simulink model "SAME5x_PIM_MCLV2_Test_programme_2020a"  (Simulink 10.1)
(part 2 of 2)

      mask TypeOptions FDMTEN: Deadman Timer is enabled | Deadman Timer is disabled
      mask TypeOptions TRCEN: Trace features in the CPU are enabled | Trace features in the CPU are disabled
      mask TypeOptions BOOTISA: Boot code and Exception code is MIPS32 | Boot code and Exception code is microMIPS
      mask TypeOptions FECCCON: ECC and Dynamic ECC are disabled (ECCCON<1:0> bits are writable) | ECC and Dynamic ECC are disabled (ECCCON<1:0> bits are locked) | Dynamic Flash ECC is enabled (ECCCON<1:0> bits are locked) | Flash ECC is enabled (ECCCON<1:0> bits are locked; disables word Flash writes) | ECC and Dynamic ECC are disabled (ECCCON bits are writable) | ECC and Dynamic ECC are disabled (ECCCON bits are locked) | Dynamic Flash ECC is enabled (ECCCON bits are locked) | Flash ECC is enabled (ECCCON bits are locked)
      mask TypeOptions EXTDDRSIZE: Not used
      mask TypeOptions FSLEEP: Flash is powered down when the device is in Sleep mode | Flash power down is controlled by the VREGS bit
      mask TypeOptions DBGPER: Allow CPU access to all permission regions | PG0: Deny PG1: Allow PG2: Allow | PG0: Allow PG1: Deny PG2: Allow | Allow CPU access to Permission Group 2 permission regions | PG0: Allow PG1: Allow PG2: Deny | Allow CPU access to Permission Group 1 permission regions | Allow CPU access to Permission Group 0 permission regions | Deny CPU access to all permission regions
      mask TypeOptions EJTAGBEN: Normal EJTAG functionality | Reduced EJTAG functionality
      mask TypeOptions TSEQ: Not used
      mask TypeOptions CSEQ: Not used
      mask TypeOptions RWDTPS: 1:1048576 | 1:524288 | 1:262144 | 1:131072 | 1:65536 | 1:32768 | 1:16384 | 1:8192 | 1:4096 | 1:2048 | 1:1024 | 1:512 | 1:256 | 1:128 | 1:64 | 1:32 | 1:16 | 1:8 | 1:4 | 1:2 | 1:1 | 1:2147483648 | 1:1073741824 | 1:536870912 | 1:268435456 | 1:134217728 | 1:67108864 | 1:33554432 | 1:16777216 | 1:8388608 | 1:4194304 | 1:2097152
      mask TypeOptions RCLKSEL: Always use LPRC | Use FRC when WINDIS = 0; system clock is not INTOSC/LPRC and device is not in Sleep;otherwise; use INTOSC/LPRC | Use peripheral clk when system clock is not INTOSC/LPRC and device is not in Sleep;otherwise; use INTOSC/LPRC | Always use BFRC/256 | Use FRC when WINDIS = 0 and device is not in Sleep; otherwise; use BFRC/256 | Use peripheral clk when device is not in Sleep; otherwise; use BFRC/256
      mask TypeOptions SWDTPS: 1:1048576 | 1:524288 | 1:262144 | 1:131072 | 1:65536 | 1:32768 | 1:16384 | 1:8192 | 1:4096 | 1:2048 | 1:1024 | 1:512 | 1:256 | 1:128 | 1:64 | 1:32 | 1:16 | 1:8 | 1:4 | 1:2 | 1:1 | 1:2147483648 | 1:1073741824 | 1:536870912 | 1:268435456 | 1:134217728 | 1:67108864 | 1:33554432 | 1:16777216 | 1:8388608 | 1:4194304 | 1:2097152
      mask TypeOptions DMTIVTL: Not used
      mask TypeOptions DMTIVTH: Not used
      mask TypeOptions DMTCNTL: Not used
      mask TypeOptions DMTCNTH: Not used
      mask TypeOptions DMTDIS: Dead Man Timer is Disabled and can be enabled by software | Dead Man Timer is Enabled and cannot be disabled by software
      mask TypeOptions SMBEN: SMBus input threshold is enabled | Standard I2C input threshold operation
      mask TypeOptions SPI2PIN: SPI2 uses I/O remap (PPS) pins | SPI2 uses dedicated I/O pins
      mask TypeOptions CTXT3: Not Assigned | Alternate Register set assigned to IPL level 7 | Alternate Register set assigned to IPL level 6 | Alternate Register set assigned to IPL level 5 | Alternate Register set assigned to IPL level 4 | Alternate Register set assigned to IPL level 3 | Alternate Register set assigned to IPL level 2 | Alternate Register set assigned to IPL level 1
      mask TypeOptions CTXT4: Not Assigned | Alternate Register set assigned to IPL level 7 | Alternate Register set assigned to IPL level 6 | Alternate Register set assigned to IPL level 5 | Alternate Register set assigned to IPL level 4 | Alternate Register set assigned to IPL level 3 | Alternate Register set assigned to IPL level 2 | Alternate Register set assigned to IPL level 1
      mask TypeOptions MBXM0: Mailbox register configured for Master data read (Slave to Master data transfer) | Mailbox register configured for Master data write (Master to Slave data transfer)
      mask TypeOptions MBXM1: Mailbox register configured for Master data read (Slave to Master data transfer) | Mailbox register configured for Master data write (Master to Slave data transfer)
      mask TypeOptions MBXM2: Mailbox register configured for Master data read (Slave to Master data transfer) | Mailbox register configured for Master data write (Master to Slave data transfer)
      mask TypeOptions MBXM3: Mailbox register configured for Master data read (Slave to Master data transfer) | Mailbox register configured for Master data write (Master to Slave data transfer)
      mask TypeOptions MBXM4: Mailbox register configured for Master data read (Slave to Master data transfer) | Mailbox register configured for Master data write (Master to Slave data transfer)
      mask TypeOptions MBXM5: Mailbox register configured for Master data read (Slave to Master data transfer) | Mailbox register configured for Master data write (Master to Slave data transfer)
      mask TypeOptions MBXM6: Mailbox register configured for Master data read (Slave to Master data transfer) | Mailbox register configured for Master data write (Master to Slave data transfer)
      mask TypeOptions MBXM7: Mailbox register configured for Master data read (Slave to Master data transfer) | Mailbox register configured for Master data write (Master to Slave data transfer)
      mask TypeOptions MBXM8: Mailbox register configured for Master data read (Slave to Master data transfer) | Mailbox register configured for Master data write (Master to Slave data transfer)
      mask TypeOptions MBXM9: Mailbox register configured for Master data read (Slave to Master data transfer) | Mailbox register configured for Master data write (Master to Slave data transfer)
      mask TypeOptions MBXM10: Mailbox register configured for Master data read (Slave to Master data transfer) | Mailbox register configured for Master data write (Master to Slave data transfer)
      mask TypeOptions MBXM11: Mailbox register configured for Master data read (Slave to Master data transfer) | Mailbox register configured for Master data write (Master to Slave data transfer)
      mask TypeOptions MBXM12: Mailbox register configured for Master data read (Slave to Master data transfer) | Mailbox register configured for Master data write (Master to Slave data transfer)
      mask TypeOptions MBXM13: Mailbox register configured for Master data read (Slave to Master data transfer) | Mailbox register configured for Master data write (Master to Slave data transfer)
      mask TypeOptions MBXM14: Mailbox register configured for Master data read (Slave to Master data transfer) | Mailbox register configured for Master data write (Master to Slave data transfer)
      mask TypeOptions MBXM15: Mailbox register configured for Master data read (Slave to Master data transfer) | Mailbox register configured for Master data write (Master to Slave data transfer)
      mask TypeOptions MBXHSA: MSIxMBXD15 assigned to mailbox handshake protocol block A | MSIxMBXD14 assigned to mailbox handshake protocol block A | MSIxMBXD13 assigned to mailbox handshake protocol block A | MSIxMBXD12 assigned to mailbox handshake protocol block A | MSIxMBXD11 assigned to mailbox handshake protocol block A | MSIxMBXD10 assigned to mailbox handshake protocol block A | MSIxMBXD9 assigned to mailbox handshake protocol block A | MSIxMBXD8 assigned to mailbox handshake protocol block A | MSIxMBXD7 assigned to mailbox handshake protocol block A | MSIxMBXD6 assigned to mailbox handshake protocol block A | MSIxMBXD5 assigned to mailbox handshake protocol block A | MSIxMBXD4 assigned to mailbox handshake protocol block A | MSIxMBXD3 assigned to mailbox handshake protocol block A | MSIxMBXD2 assigned to mailbox handshake protocol block A | MSIxMBXD1 assigned to mailbox handshake protocol block A | MSIxMBXD0 assigned to mailbox handshake protocol block A
      mask TypeOptions MBXHSB: MSIxMBXD15 assigned to mailbox handshake protocol block B | MSIxMBXD14 assigned to mailbox handshake protocol block B | MSIxMBXD13 assigned to mailbox handshake protocol block B | MSIxMBXD12 assigned to mailbox handshake protocol block B | MSIxMBXD11 assigned to mailbox handshake protocol block B | MSIxMBXD10 assigned to mailbox handshake protocol block B | MSIxMBXD9 assigned to mailbox handshake protocol block B | MSIxMBXD8 assigned to mailbox handshake protocol block B | MSIxMBXD7 assigned to mailbox handshake protocol block B | MSIxMBXD6 assigned to mailbox handshake protocol block B | MSIxMBXD5 assigned to mailbox handshake protocol block B | MSIxMBXD4 assigned to mailbox handshake protocol block B | MSIxMBXD3 assigned to mailbox handshake protocol block B | MSIxMBXD2 assigned to mailbox handshake protocol block B | MSIxMBXD1 assigned to mailbox handshake protocol block B | MSIxMBXD0 assigned to mailbox handshake protocol block B
      mask TypeOptions MBXHSC: MSIxMBXD15 assigned to mailbox handshake protocol block C | MSIxMBXD14 assigned to mailbox handshake protocol block C | MSIxMBXD13 assigned to mailbox handshake protocol block C | MSIxMBXD12 assigned to mailbox handshake protocol block C | MSIxMBXD11 assigned to mailbox handshake protocol block C | MSIxMBXD10 assigned to mailbox handshake protocol block C | MSIxMBXD9 assigned to mailbox handshake protocol block C | MSIxMBXD8 assigned to mailbox handshake protocol block C | MSIxMBXD7 assigned to mailbox handshake protocol block C | MSIxMBXD6 assigned to mailbox handshake protocol block C | MSIxMBXD5 assigned to mailbox handshake protocol block C | MSIxMBXD4 assigned to mailbox handshake protocol block C | MSIxMBXD3 assigned to mailbox handshake protocol block C | MSIxMBXD2 assigned to mailbox handshake protocol block C | MSIxMBXD1 assigned to mailbox handshake protocol block C | MSIxMBXD0 assigned to mailbox handshake protocol block C
      mask TypeOptions MBXHSD: MSIxMBXD15 assigned to mailbox handshake protocol block D | MSIxMBXD14 assigned to mailbox handshake protocol block D | MSIxMBXD13 assigned to mailbox handshake protocol block D | MSIxMBXD12 assigned to mailbox handshake protocol block D | MSIxMBXD11 assigned to mailbox handshake protocol block D | MSIxMBXD10 assigned to mailbox handshake protocol block D | MSIxMBXD9 assigned to mailbox handshake protocol block D | MSIxMBXD8 assigned to mailbox handshake protocol block D | MSIxMBXD7 assigned to mailbox handshake protocol block D | MSIxMBXD6 assigned to mailbox handshake protocol block D | MSIxMBXD5 assigned to mailbox handshake protocol block D | MSIxMBXD4 assigned to mailbox handshake protocol block D | MSIxMBXD3 assigned to mailbox handshake protocol block D | MSIxMBXD2 assigned to mailbox handshake protocol block D | MSIxMBXD1 assigned to mailbox handshake protocol block D | MSIxMBXD0 assigned to mailbox handshake protocol block D
      mask TypeOptions MBXHSE: MSIxMBXD15 assigned to mailbox handshake protocol block E | MSIxMBXD14 assigned to mailbox handshake protocol block E | MSIxMBXD13 assigned to mailbox handshake protocol block E | MSIxMBXD12 assigned to mailbox handshake protocol block E | MSIxMBXD11 assigned to mailbox handshake protocol block E | MSIxMBXD10 assigned to mailbox handshake protocol block E | MSIxMBXD9 assigned to mailbox handshake protocol block E | MSIxMBXD8 assigned to mailbox handshake protocol block E | MSIxMBXD7 assigned to mailbox handshake protocol block E | MSIxMBXD6 assigned to mailbox handshake protocol block E | MSIxMBXD5 assigned to mailbox handshake protocol block E | MSIxMBXD4 assigned to mailbox handshake protocol block E | MSIxMBXD3 assigned to mailbox handshake protocol block E | MSIxMBXD2 assigned to mailbox handshake protocol block E | MSIxMBXD1 assigned to mailbox handshake protocol block E | MSIxMBXD0 assigned to mailbox handshake protocol block E
      mask TypeOptions MBXHSF: MSIxMBXD15 assigned to mailbox handshake protocol block F | MSIxMBXD14 assigned to mailbox handshake protocol block F | MSIxMBXD13 assigned to mailbox handshake protocol block F | MSIxMBXD12 assigned to mailbox handshake protocol block F | MSIxMBXD11 assigned to mailbox handshake protocol block F | MSIxMBXD10 assigned to mailbox handshake protocol block F | MSIxMBXD9 assigned to mailbox handshake protocol block F | MSIxMBXD8 assigned to mailbox handshake protocol block F | MSIxMBXD7 assigned to mailbox handshake protocol block F | MSIxMBXD6 assigned to mailbox handshake protocol block F | MSIxMBXD5 assigned to mailbox handshake protocol block F | MSIxMBXD4 assigned to mailbox handshake protocol block F | MSIxMBXD3 assigned to mailbox handshake protocol block F | MSIxMBXD2 assigned to mailbox handshake protocol block F | MSIxMBXD1 assigned to mailbox handshake protocol block F | MSIxMBXD0 assigned to mailbox handshake protocol block F
      mask TypeOptions MBXHSG: MSIxMBXD15 assigned to mailbox handshake protocol block G | MSIxMBXD14 assigned to mailbox handshake protocol block G | MSIxMBXD13 assigned to mailbox handshake protocol block G | MSIxMBXD12 assigned to mailbox handshake protocol block G | MSIxMBXD11 assigned to mailbox handshake protocol block G | MSIxMBXD10 assigned to mailbox handshake protocol block G | MSIxMBXD9 assigned to mailbox handshake protocol block G | MSIxMBXD8 assigned to mailbox handshake protocol block G | MSIxMBXD7 assigned to mailbox handshake protocol block G | MSIxMBXD6 assigned to mailbox handshake protocol block G | MSIxMBXD5 assigned to mailbox handshake protocol block G | MSIxMBXD4 assigned to mailbox handshake protocol block G | MSIxMBXD3 assigned to mailbox handshake protocol block G | MSIxMBXD2 assigned to mailbox handshake protocol block G | MSIxMBXD1 assigned to mailbox handshake protocol block G | MSIxMBXD0 assigned to mailbox handshake protocol block G
      mask TypeOptions MBXHSH: MSIxMBXD15 assigned to mailbox handshake protocol block H | MSIxMBXD14 assigned to mailbox handshake protocol block H | MSIxMBXD13 assigned to mailbox handshake protocol block H | MSIxMBXD12 assigned to mailbox handshake protocol block H | MSIxMBXD11 assigned to mailbox handshake protocol block H | MSIxMBXD10 assigned to mailbox handshake protocol block H | MSIxMBXD9 assigned to mailbox handshake protocol block H | MSIxMBXD8 assigned to mailbox handshake protocol block H | MSIxMBXD7 assigned to mailbox handshake protocol block H | MSIxMBXD6 assigned to mailbox handshake protocol block H | MSIxMBXD5 assigned to mailbox handshake protocol block H | MSIxMBXD4 assigned to mailbox handshake protocol block H | MSIxMBXD3 assigned to mailbox handshake protocol block H | MSIxMBXD2 assigned to mailbox handshake protocol block H | MSIxMBXD1 assigned to mailbox handshake protocol block H | MSIxMBXD0 assigned to mailbox handshake protocol block H
      mask TypeOptions HSAEN: Mailbox data flow control handshake protocol block disabled. | Mailbox data flow control handshake protocol block enabled
      mask TypeOptions HSBEN: Mailbox data flow control handshake protocol block disabled. | Mailbox data flow control handshake protocol block enabled
      mask TypeOptions HSCEN: Mailbox data flow control handshake protocol block disabled. | Mailbox data flow control handshake protocol block enabled
      mask TypeOptions HSDEN: Mailbox data flow control handshake protocol block disabled. | Mailbox data flow control handshake protocol block enabled
      mask TypeOptions HSEEN: Mailbox data flow control handshake protocol block disabled. | Mailbox data flow control handshake protocol block enabled
      mask TypeOptions HSFEN: Mailbox data flow control handshake protocol block disabled. | Mailbox data flow control handshake protocol block enabled
      mask TypeOptions HSGEN: Mailbox data flow control handshake protocol block disabled. | Mailbox data flow control handshake protocol block enabled
      mask TypeOptions HSHEN: Mailbox data flow control handshake protocol block disabled. | Mailbox data flow control handshake protocol block enabled
      mask TypeOptions CPRA0: Master core owns pin. | Slave 1 core owns pin.
      mask TypeOptions CPRA1: Master core owns pin. | Slave 1 core owns pin.
      mask TypeOptions CPRA2: Master core owns pin. | Slave 1 core owns pin.
      mask TypeOptions CPRA3: Master core owns pin. | Slave 1 core owns pin.
      mask TypeOptions CPRA4: Master core owns pin. | Slave 1 core owns pin.
      mask TypeOptions CPRB0: Master core owns pin. | Slave 1 core owns pin.
      mask TypeOptions CPRB1: Master core owns pin. | Slave 1 core owns pin.
      mask TypeOptions CPRB2: Master core owns pin. | Slave 1 core owns pin.
      mask TypeOptions CPRB3: Master core owns pin. | Slave 1 core owns pin.
      mask TypeOptions CPRB4: Master core owns pin. | Slave 1 core owns pin.
      mask TypeOptions CPRB5: Master core owns pin. | Slave 1 core owns pin.
      mask TypeOptions CPRB6: Master core owns pin. | Slave 1 core owns pin.
      mask TypeOptions CPRB7: Master core owns pin. | Slave 1 core owns pin.
      mask TypeOptions CPRB8: Master core owns pin. | Slave 1 core owns pin.
      mask TypeOptions CPRB9: Master core owns pin. | Slave 1 core owns pin.
      mask TypeOptions CPRB10: Master core owns pin. | Slave 1 core owns pin.
      mask TypeOptions CPRB11: Master core owns pin. | Slave 1 core owns pin.
      mask TypeOptions CPRB12: Master core owns pin. | Slave 1 core owns pin.
      mask TypeOptions CPRB13: Master core owns pin. | Slave 1 core owns pin.
      mask TypeOptions CPRB14: Master core owns pin. | Slave 1 core owns pin.
      mask TypeOptions CPRB15: Master core owns pin. | Slave 1 core owns pin.
      mask TypeOptions CPRC0: Master core owns pin. | Slave 1 core owns pin.
      mask TypeOptions CPRC1: Master core owns pin. | Slave 1 core owns pin.
      mask TypeOptions CPRC2: Master core owns pin. | Slave 1 core owns pin.
      mask TypeOptions CPRC3: Master core owns pin. | Slave 1 core owns pin.
      mask TypeOptions CPRC4: Master core owns pin. | Slave 1 core owns pin.
      mask TypeOptions CPRC5: Master core owns pin. | Slave 1 core owns pin.
      mask TypeOptions CPRC6: Master core owns pin. | Slave 1 core owns pin.
      mask TypeOptions CPRC7: Master core owns pin. | Slave 1 core owns pin.
      mask TypeOptions CPRC8: Master core owns pin. | Slave 1 core owns pin.
      mask TypeOptions CPRC9: Master core owns pin. | Slave 1 core owns pin.
      mask TypeOptions CPRC10: Master core owns pin. | Slave 1 core owns pin.
      mask TypeOptions CPRC11: Master core owns pin. | Slave 1 core owns pin.
      mask TypeOptions CPRC12: Master core owns pin. | Slave 1 core owns pin.
      mask TypeOptions CPRC13: Master core owns pin. | Slave 1 core owns pin.
      mask TypeOptions CPRC14: Master core owns pin. | Slave 1 core owns pin.
      mask TypeOptions CPRC15: Master core owns pin. | Slave 1 core owns pin.
      mask TypeOptions CPRD0: Master core owns pin. | Slave 1 core owns pin.
      mask TypeOptions CPRD1: Master core owns pin. | Slave 1 core owns pin.
      mask TypeOptions CPRD2: Master core owns pin. | Slave 1 core owns pin.
      mask TypeOptions CPRD3: Master core owns pin. | Slave 1 core owns pin.
      mask TypeOptions CPRD4: Master core owns pin. | Slave 1 core owns pin.
      mask TypeOptions CPRD5: Master core owns pin. | Slave 1 core owns pin.
      mask TypeOptions CPRD6: Master core owns pin. | Slave 1 core owns pin.
      mask TypeOptions CPRD7: Master core owns pin. | Slave 1 core owns pin.
      mask TypeOptions CPRD8: Master core owns pin. | Slave 1 core owns pin.
      mask TypeOptions CPRD9: Master core owns pin. | Slave 1 core owns pin.
      mask TypeOptions CPRD10: Master core owns pin. | Slave 1 core owns pin.
      mask TypeOptions CPRD11: Master core owns pin. | Slave 1 core owns pin.
      mask TypeOptions CPRD12: Master core owns pin. | Slave 1 core owns pin.
      mask TypeOptions CPRD13: Master core owns pin. | Slave 1 core owns pin.
      mask TypeOptions CPRD14: Master core owns pin. | Slave 1 core owns pin.
      mask TypeOptions CPRD15: Master core owns pin. | Slave 1 core owns pin.
      mask TypeOptions CPRE0: Master core owns pin. | Slave 1 core owns pin.
      mask TypeOptions CPRE1: Master core owns pin. | Slave 1 core owns pin.
      mask TypeOptions CPRE2: Master core owns pin. | Slave 1 core owns pin.
      mask TypeOptions CPRE3: Master core owns pin. | Slave 1 core owns pin.
      mask TypeOptions CPRE4: Master core owns pin. | Slave 1 core owns pin.
      mask TypeOptions CPRE5: Master core owns pin. | Slave 1 core owns pin.
      mask TypeOptions CPRE6: Master core owns pin. | Slave 1 core owns pin.
      mask TypeOptions CPRE7: Master core owns pin. | Slave 1 core owns pin.
      mask TypeOptions CPRE8: Master core owns pin. | Slave 1 core owns pin.
      mask TypeOptions CPRE9: Master core owns pin. | Slave 1 core owns pin.
      mask TypeOptions CPRE10: Master core owns pin. | Slave 1 core owns pin.
      mask TypeOptions CPRE11: Master core owns pin. | Slave 1 core owns pin.
      mask TypeOptions CPRE12: Master core owns pin. | Slave 1 core owns pin.
      mask TypeOptions CPRE13: Master core owns pin. | Slave 1 core owns pin.
      mask TypeOptions CPRE14: Master core owns pin. | Slave 1 core owns pin.
      mask TypeOptions CPRE15: Master core owns pin. | Slave 1 core owns pin.
      mask TypeOptions S1FNOSC: Internal Fast RC (FRC) Oscillator with postscaler | Back up Fast RC (BFRC) Oscillator | Low-Power RC Oscillator (LPRC) | Primary Oscillator with PLL module (XT + PLL; HS + PLL; EC + PLL) | Primary Oscillator (XT; HS; EC) | Fast RC Oscillator with divide-by-N with PLL module (FRCPLL)  | Internal Fast RC (FRC)
      mask TypeOptions S1IESO: Start up with FRC; then switch | Disable
      mask TypeOptions S1OSCIOFNC: OSC2 is clock output | general purpose digital I/O pin
      mask TypeOptions S1FCKSM: Both Clock switching and Fail-safe Clock Monitor are disabled | Clock switching is enabled;Fail-safe Clock Monitor is disabled | Both Clock switching and Fail-safe Clock Monitor are enabled
      mask TypeOptions S1PLLKEN: S1PLLKEN_ON | S1PLLKEN_OFF
      mask TypeOptions S1RWDTPS: 1:1048576 | 1:524288 | 1:262144 | 1:131072 | 1:65536 | 1:32768 | 1:16384 | 1:8192 | 1:4096 | 1:2048 | 1:1024 | 1:512 | 1:256 | 1:128 | 1:64 | 1:32 | 1:16 | 1:8 | 1:4 | 1:2 | 1:1
      mask TypeOptions S1RCLKSEL: Always use LPRC | Use FRC when WINDIS = 0; system clock is not INTOSC/LPRC and device is not in Sleep; otherwise; use INTOSC/LPRC | Use peripheral clk when system clock is not INTOSC/LPRC and device is not in Sleep;otherwise; use INTOSC/LPRC
      mask TypeOptions S1WINDIS: Watchdog Timer operates in Non-Window mode | Watchdog Timer operates in Window mode
      mask TypeOptions S1WDTWIN: WDT Window is 25% of WDT period | WDT Window is 37.5% of WDT period | WDT Window is 50% of WDT period | WDT Windo is 75% of WDT period
      mask TypeOptions S1SWDTPS: 1:1048576 | 1:524288 | 1:262144 | 1:131072 | 1:65536 | 1:32768 | 1:16384 | 1:8192 | 1:4096 | 1:2048 | 1:1024 | 1:512 | 1:256 | 1:128 | 1:64 | 1:32 | 1:16 | 1:8 | 1:4 | 1:2 | 1:1
      mask TypeOptions S1FWDTEN: Enable | Disable
      mask TypeOptions S1ICS: Communicate on PGC1 and PGD1 | Communicate on PGC2 and PGD2 | Communicate on PGC3 and PGD3
      mask TypeOptions S1DEBUG: Not used
      mask TypeOptions S1ISOLAT: The slave can operate (in debug mode) even if the SLVEN bit in the MSI is zero. | The slave can only operate if the SLVEN bit in the MSI is set.
      mask TypeOptions S1NOBTSWP: BOOTSWP instruction is disabled | BOOTSWP instruction is enabled
      mask TypeOptions S1ALTI2C1: I2C1 mapped to SDA1/SCL1 pins | I2C1 mapped to ASDA1/ASCL1 pins
      mask TypeOptions S1SPI1PIN: Slave SPI1 uses I/O remap (PPS) pins | Slave SPI1 uses dedicated I/O pins
      mask TypeOptions S1SSRE: Slave generated resets will reset the Slave Enable Bit in the MSI module | Slave generated resets will not reset the Slave Enable Bit in the MSI module
      mask TypeOptions S1MSRE: The master software oriented RESET events (RESET Op-Code; Watchdog timeout; TRAP reset; illegalInstruction) will also cause the slave subsystem to reset. | The master software oriented RESET events (RESET Op-Code; Watchdog timeout; TRAP reset; illegalInstruction) will not cause the slave subsystem to reset.
      mask TypeOptions S1CTXT1: Not Assigned | Alternate Register set assigned to IPL level 7 | Alternate Register set assigned to IPL level 6 | Alternate Register set assigned to IPL level 5 | Alternate Register set assigned to IPL level 4 | Alternate Register set assigned to IPL level 3 | Alternate Register set assigned to IPL level 2 | Alternate Register set assigned to IPL level 1
      mask TypeOptions S1CTXT2: Not Assigned | Alternate Register set assigned to IPL level 7 | Alternate Register set assigned to IPL level 6 | Alternate Register set assigned to IPL level 5 | Alternate Register set assigned to IPL level 4 | Alternate Register set assigned to IPL level 3 | Alternate Register set assigned to IPL level 2 | Alternate Register set assigned to IPL level 1
      mask TypeOptions S1CTXT3: Not Assigned | Alternate Register set assigned to IPL level 7 | Alternate Register set assigned to IPL level 6 | Alternate Register set assigned to IPL level 5 | Alternate Register set assigned to IPL level 4 | Alternate Register set assigned to IPL level 3 | Alternate Register set assigned to IPL level 2 | Alternate Register set assigned to IPL level 1
      mask TypeOptions S1CTXT4: Not Assigned | Alternate Register set assigned to IPL level 7 | Alternate Register set assigned to IPL level 6 | Alternate Register set assigned to IPL level 5 | Alternate Register set assigned to IPL level 4 | Alternate Register set assigned to IPL level 3 | Alternate Register set assigned to IPL level 2 | Alternate Register set assigned to IPL level 1
      mask TypeOptions BORLVL: Not used
      mask TypeOptions BSSO: Not used
      mask TypeOptions MCA: Not used
      mask TypeOptions MAXTEMP: Not used
      mask TypeOptions CFGAN14: Not used
      mask TypeOptions CFGAN15: Not used
      mask TypeOptions S1IOL1WAY: Not used
      mask TypeOptions S1BSSO: Not used
      mask TypeOptions S1BACKBUG: Not used
      mask TypeOptions BISTDIS: mBIST on reset feature disabled | mBIST on reset feature enabled
      mask TypeOptions NOBTSWP: BOOTSWP instruction is disabled | BOOTSWP instruction is enabled
      mask TypeOptions S1BISTDIS: Slave BIST on reset feature disabled | Slave BIST on reset feature enabled
      mask TypeOptions S1DMTIVTL: Not used
      mask TypeOptions S1DMTIVTH: Not used
      mask TypeOptions S1DMTCNTL: Not used
      mask TypeOptions S1DMTCNTH: Not used
      mask TypeOptions S1DMTDIS: Slave Dead Man Timer is Disabled and can be enabled by software | Slave Dead Man Timer is Enabled and cannot be disabled by software
      mask TypeOptions BSEQ: Not used
      mask TypeOptions IBSEQ: Not used
      mask TypeOptions SMB3EN: SMBus 3.0 input levels | Normal  SMBus input levels
      mask TypeOptions FUSBIDIO2: USBID pin is controlled by the USB2 module | USBID pin is controlled by the port function
      mask TypeOptions FVBUSIO2: VBUSON pin is controlled by the USB2 module | VBUSON pin is controlled by the port function
      mask TypeOptions FUSBIDIO1: USBID pin is controlled by the USB1 module | USBID pin is controlled by the port function
      mask TypeOptions FVBUSIO1: VBUSON pin is controlled by the USB1 module | VBUSON pin is controlled by the port function
      mask TypeOptions VBATBOREN: Enable ZPBOR during VBAT Mode | Disable ZPBOR during VBAT Mode
      mask TypeOptions FDSEN: Enable DSEN bit in DSCON | Disable DSEN bit in DSCON
      mask TypeOptions BORSEL: BOR trip voltage 2.1v (Non-OPAMP deviced operation) | BOR trip voltage 2.8v (OPAMP deviced operation)
      mask TypeOptions POSCFGAIN: Gain is G3 | Gain is G2 | Gain is G1 | Gain is G0
      mask TypeOptions POSCAGCDLY: Settling time = 25ms x AGCRNG | Settling time = 6.25ms x AGCRNG | Settling time = 400ms x AGCRNG | Settling time = 100ms x AGCRNG
      mask TypeOptions POSCAGCRNG: Range 1x | Range 5x
      mask TypeOptions POSCAGC: Automatic Gain Control for Oscillator | Manual Gain Control of Oscillator
      mask TypeOptions FDBGWP: Not used
      mask Display: MCHP_DrawLogo;fprintf('MCHP_MASTER\\nSAME54P20A - TQFP128\\n100MHZ');
  Model Info : simulink/Model-Wide Utilities/Model Info  Frame=on  DisplayStringWithTags=|  HorizontalTextAlignment=Center  LeftAlignmentValue=0.5
      | %<ModelName> v%<ModelVersion> - %<Creator>
      | 
      | %<Description>
      | 
      | Last modified on: %<LastModificationDate>
  Port Info : S-Function  FunctionName=MCHP_EmptySFunction  SFunctionDeploymentMode=off  EnableBusSupport=off  mask{MCHP_MASTERLINK=SAME5x_PIM_MCLV2_Test_programme/Microchip Master}
      mask init:
      | MCHP_PortInfo_Callback(gcbh,'INITIALISATION');
      settings: CopyFcn=MCHP_PortInfo_Callback(gcb,'COPY');  OpenFcn=MCHP_PortInfo_Callback(gcb,'OPEN');
      mask Display: MCHP_DrawLogo;text(.05,20,'[Pin]  Port   -  Desc\n[102]   PB26 -  DOU -  ( Digital Out )','verticalalignment','Top','horizontalalignment','left');text(.95,0.05,'(1 pins)','verticalalignment','Bottom','horizontalalignment','right');
  wires:
  Counter Limited/1 -> Data Type Conversion/1  "U2 CH1"
  Data Type Conversion/1 -> DBG_LED2/1
